simulink model "RR_Target_sim"  (R2023b)
settings: Solver=VariableStepAuto  StartTime=0.0  StopTime=100  RelTol=1e-3
values from neighbouring files (symbols this model uses):
  RR_Aero_Aoa = [-40 -20 -10 -5 0 5 10 20 40]    [RR.mat]    (also in aero.m = [-40.0, -20.0, -10.0, -5.0, 0.0, 5.0, 10.0, 20.0, 40.0])
  RR_Aero_CD = [0.682566420597 0.618503123563 0.559439658146 0.524132967178 0.485737326161 0.447874599784 0.410140259349 0.344355457301 0.271986762452 0.285740001736 0.220860646778 0.173194791928 ... (405 elements, 9x9x5)]    [RR.mat]    (also in aero.m = flip([0.271986762452 0.048967807354 0.024623797928 0.0311930)
  RR_Aero_CL = [-1.32787481318 -1.28000797148 -1.22978921447 -1.19580936529 -1.15925228344 -1.11732991534 -1.07321949156 -0.982213833372 -0.840672452343 -1.01110225062 -0.901800471345 -0.804191382013 ... (405 elements, 9x9x5)]    [RR.mat]    (also in aero.m = flip([-0.840672452343 -0.271053660865 0.064194032020 0.23384)
  RR_Aero_CMy = [0.261776710059 0.227892723507 0.194122810948 0.17203964717 0.149197278338 0.123782621534 0.09809104025 0.048156954183 -0.022673613914 0.230490752369 0.172298182326 0.122095577928 ... (405 elements, 9x9x5)]    [RR.mat]    (also in aero.m = flip([-0.022673613914 -0.123256713392 -0.153636001960 -0.164)
  RR_Aero_Elevons = [-40 -20 -10 -5 0 5 10 20 40]    [RR.mat]    (also in aero.m = [-40.0, -20.0, -10.0, -5.0, 0.0, 5.0, 10.0, 20.0, 40.0])
  RR_Aero_Mach = [0.01 0.1 0.2 0.5 0.9]    [RR.mat]    (also in aero.m = [0.01, 0.1, 0.2, 0.5, 0.9])
  RR_Iyy = 4.432    [RR.mat]
  RR_Motors_Thrust = [4.04656097579 98.9159349639]    [RR.mat]
  RR_Motors_Thrust_Alt_Lut = [0 10000 20000 30000]    [RR.mat]
  RR_Motors_Thrust_Pct_Lut = [1 0.705882352941 0.470588235294 0.352941176471]    [RR.mat]
  RR_Span = 3.6    [RR.mat]
  RR_X_CG = 0.732425    [RR.mat]
  RR_X_NP = 0.9170209    [RR.mat]
  SIM_G = 32.174    [RR.mat]    (also in RR_Forces_ws.m = G; RR_Pitch_ws.m = G; RR_Target_sim_ws.m = G; RR_Target_ws.m = G)
  SIM_INITAL_ALT = -1000    [RR.mat]    (also in RR_Forces_ws.m; RR_Pitch_ws.m = 0; RR_Target_sim_ws.m = 0; RR_Target_ws.m = 0)
  SIM_INITAL_PITCH = 90    [RR_Target_sim_ws.m]    (also in RR_Target_ws.m)
  SIM_INITAL_VEL = 750    [RR.mat]    (also in RR_Forces_ws.m; RR_Pitch_ws.m = 11; RR_Target_sim_ws.m = 15; RR_Target_ws.m = 15)
  SIM_TARGET_ALT = -20000    [RR_Target_sim_ws.m]    (also in RR_Target_ws.m)
  SIM_TARGET_VEL = convvel(290,'kts','ft/s')    [RR_Target_sim_ws.m]    (also in RR_Target_ws.m)
  SIM_TARGET_X = 10    [RR_Target_sim_ws.m]    (also in RR_Target_ws.m = 5000)
undefined symbols (not defined in the file or in its folder): deg, rad, s
libraries: simulink_extras x4, aerolibasang x2, simulink x1, slpidlib x1, aerolib6dof2 x1, aerolibconvert2 x1, aerolibadyn x1, aerolibatmos2 x1, aerolibguid x1, vrlib x1
settings Model: Creator=jrighetti  LastModifiedBy=jrighetti

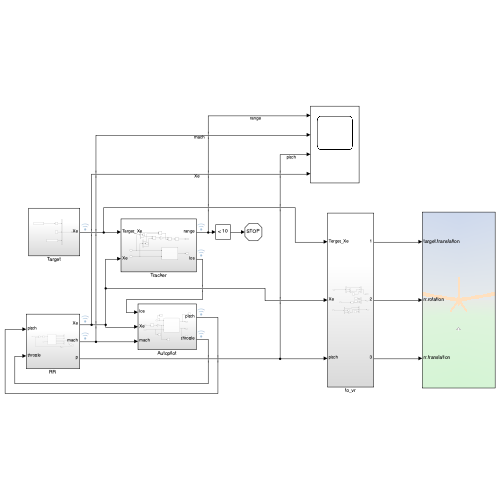
[thumbnail: Simulink's stored preview of the top-level diagram]
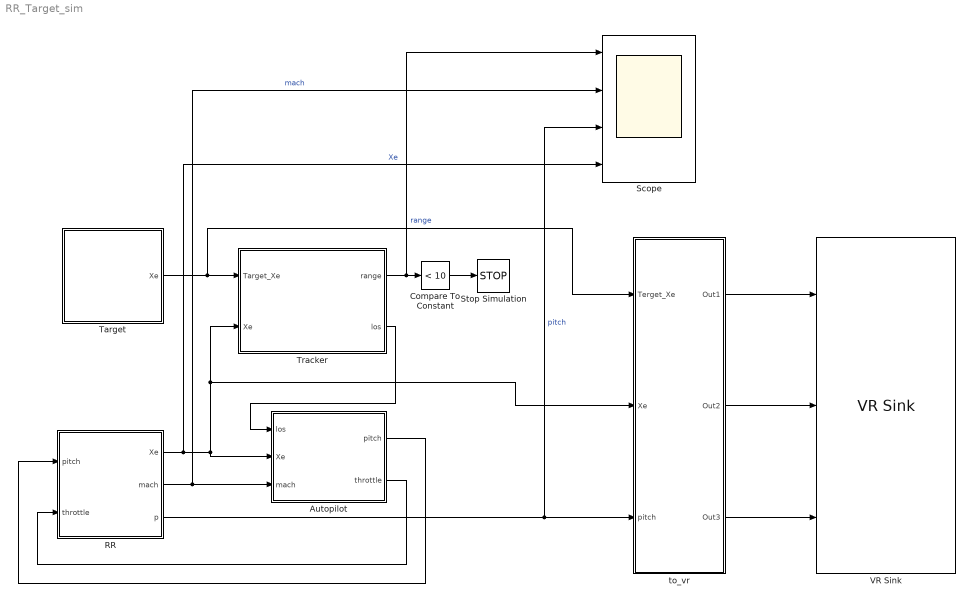
== system RR_Target_sim ==
  Autopilot : Subsystem
  Compare To Constant : simulink/Logic and Bit Operations/Compare To Constant  relop=<  const=10  OutDataTypeStr=boolean
  RR : Subsystem
  Scope : Scope  NumInputPorts=4
  Stop Simulation : Stop
  Target : Subsystem
  Tracker : Subsystem
  VR Sink : vrlib/VR Sink  InstantiateOnLoad=on  SampleTime=-1  ViewEnable=on  RemoteChange=off  RemoteView=off  FieldsWritten=target.translation.3.1.1.double#rr.rotation.4.1.1.double#rr.translation.3.1.1.double  WorldFileName=RR_Target_sim.x3d  AutoView=on  VideoDimensions=[]  AllowVariableSize=off
  to_vr : Subsystem
  wires:
  Target/1(Xe) -> to_vr/1(Terget_Xe), Tracker/1(Target_Xe)
  Compare To Constant/1 -> Stop Simulation/1
  Tracker/1(range) -> Scope/1, Compare To Constant/1  "range"
  RR/1(Xe) -> Scope/4, to_vr/2(Xe), Tracker/2(Xe), Autopilot/2(Xe)  "Xe"
  Tracker/2(los) -> Autopilot/1(los)
  RR/2(mach) -> Scope/2, Autopilot/3(mach)  "mach"
  Autopilot/1(pitch) -> RR/1(pitch)
  Autopilot/2(throttle) -> RR/2(throttle)
  RR/3(p) -> Scope/3, to_vr/3(pitch)  "pitch"
  to_vr/1(Out1) -> VR Sink/1
  to_vr/2(Out2) -> VR Sink/2
  to_vr/3(Out3) -> VR Sink/3

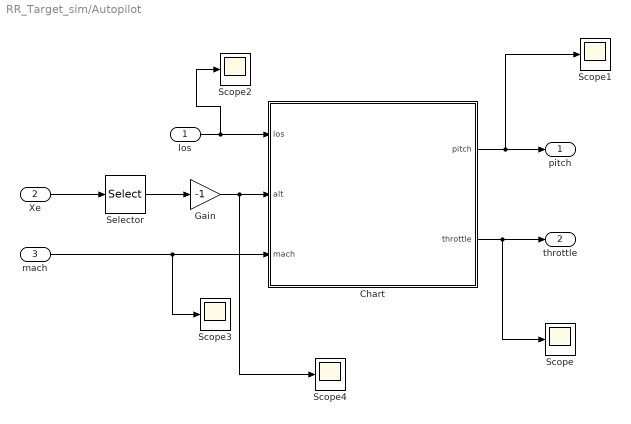
== system RR_Target_sim/Autopilot ==
  los : Inport
  Xe : Inport  Port=2
  mach : Inport  Port=3
  Chart : Stateflow chart  TreatAsAtomicUnit=on
  Gain : Gain  Gain=-1
  Scope{,1..4} (5 alike) : Scope
  Selector : Selector  InputPortWidth=3  IndexOptions=Index vector (dialog)  Indices=3  OutputSizes=1
  pitch : Outport
  throttle : Outport  Port=2
  wires:
  los/1 -> Scope2/1, Chart/1(los)
  Xe/1 -> Selector/1
  mach/1 -> Scope3/1, Chart/3(mach)
  Chart/2(throttle) -> Scope/1, throttle/1
  Selector/1 -> Gain/1
  Gain/1 -> Scope4/1, Chart/2(alt)
  Chart/1(pitch) -> Scope1/1, pitch/1

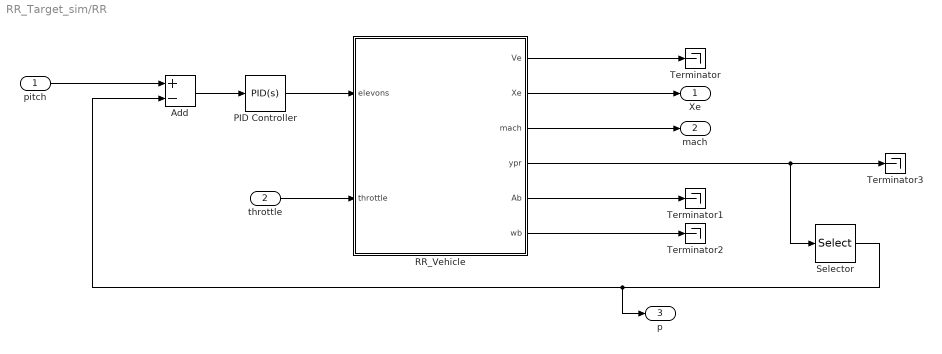
== system RR_Target_sim/RR ==
  pitch : Inport
  throttle : Inport  Port=2
  Add : Sum  Inputs=+-
  PID Controller : slpidlib/PID Controller  Controller=PID  Form=Parallel  TimeDomain=Continuous-time  UseExternalTs=off  SampleTime=-1  IntegratorMethod=Forward Euler  FilterMethod=Forward Euler  ControllerParametersSource=internal  P=0.454470686879052  I=0.32028398620468  UseKiTs=off  D=0.0230057100877012  N=14.587296267084  UseFilter=on  TunerSelectOption=Transfer Function Based (PID Tuner App)  InitialConditionSource=internal  InitialConditionForIntegrator=0  InitialConditionForFilter=0  DifferentiatorICPrevScaledInput=0  ExternalReset=none  TrackingMode=off  Kt=1  LimitOutput=off  SatLimitsSource=internal  UpperSaturationLimit=inf  LowerSaturationLimit=-inf  LinearizeAsGain=on  AntiWindupMode=none  Kb=1  LimitIntegrator=off  UpperIntegratorSaturationLimit=inf  LowerIntegratorSaturationLimit=-inf  POutMin=[]  POutMax=[]  IOutMin=[]  IOutMax=[]  DOutMin=[]  DOutMax=[]  NOutMin=[]  NOutMax=[]  SumOutMin=[]  SumOutMax=[]  SaturationOutMin=[]  SaturationOutMax=[]  PParamMin=[]  PParamMax=[]  IParamMin=[]  IParamMax=[]  DParamMin=[]  DParamMax=[]  NParamMin=[]  NParamMax=[]  KbParamMin=[]  KbParamMax=[]  KtParamMin=[]  KtParamMax=[]  KbOutMin=[]  KbOutMax=[]  KtOutMin=[]  KtOutMax=[]  IntegratorOutMin=[]  IntegratorOutMax=[]  FilterOutMin=[]  FilterOutMax=[]  SumI1OutMin=[]  SumI1OutMax=[]  SumI2OutMin=[]  SumI2OutMax=[]  SumI3OutMin=[]  SumI3OutMax=[]  SumI4OutMin=[]  SumI4OutMax=[]  SumDOutMin=[]  SumDOutMax=[]  DifferentiatorOutMin=[]  DifferentiatorOutMax=[]  FilterDiffOutCoefMin=[]  FilterDiffOutCoefMax=[]  ReciprocalOutMin=[]  ReciprocalOutMax=[]  SumDenOutMin=[]  SumDenOutMax=[]  SumNumOutMin=[]  SumNumOutMax=[]  DivideOutMin=[]  DivideOutMax=[]  UdiffTsProdOutMin=[]  UdiffTsProdOutMax=[]  NTsProdOutMin=[]  NTsProdOutMax=[]  UintegralTsProdOutMin=[]  UintegralTsProdOutMax=[]  UngainTsProdOutMin=[]  UngainTsProdOutMax=[]  ClampingZeroOutDataTypeStr=Inherit: Inherit via back propagation  ClampingZeroOutMin=[]  ClampingZeroOutMax=[]  FilterDenConstantOutDataTypeStr=Inherit: Inherit via back propagation  FilterDenConstantOutMin=[]  FilterDenConstantOutMax=[]  PCopyOutDataTypeStr=Inherit: Inherit via back propagation  PCopyOutMin=[]  PCopyOutMax=[]  NCopyOutDataTypeStr=Inherit: Inherit via back propagation  NCopyOutMin=[]  NCopyOutMax=[]  IntegratorContinuousStateAttributes=''  IntegratorStateMustResolveToSignalObject=off  IntegratorRTWStateStorageClass=Auto  FilterContinuousStateAttributes=''  FilterStateMustResolveToSignalObject=off  FilterRTWStateStorageClass=Auto  ParallelPVariant=InternalParameters  IdealPVariant=Disabled  IVariant=InternalParameters  DVariant=InternalParameters  IntegratorVariant=Continuous  SatVariant=Disabled  AWVariant=Passthrough  PCopyVariant=Disabled  TRVariant=Disabled  FdbkBlocksVariant=Forward  IdealPFdbkVariant=Disabled  SatFdbkVariant=Disabled  DerivativeFilterVariant=ContFilter  NVariant=InternalParameters  NCopyVariant=Disabled  FilterICVariant=InternalICsFilter  IntegratorICVariant=InternalICs  ExternalResetVariant=Disabled  TRSumVariant=Passthrough  SumFdbkVariant=Disabled  SumVariant=Sum_PID  TsampFilterVariant=InternalTs  TsampNgainVariant=Passthrough  TsampIntegralVariant=Disabled_SignalSpec  ExternalSaturationOutDataTypeStr=Inherit: Same as second input
  RR_Vehicle : Subsystem
  Selector : Selector  InputPortWidth=3  IndexOptions=Index vector (dialog)  Indices=2  OutputSizes=1
  Terminator{,1..3} (4 alike) : Terminator
  Xe : Outport
  mach : Outport  Port=2
  p : Outport  Port=3
  wires:
  RR_Vehicle/2(Xe) -> Xe/1
  pitch/1 -> Add/1
  PID Controller/1 -> RR_Vehicle/1(elevons)
  Selector/1 -> p/1, Add/2
  RR_Vehicle/4(ypr) -> Terminator3/1, Selector/1
  RR_Vehicle/6(wb) -> Terminator2/1
  RR_Vehicle/5(Ab) -> Terminator1/1
  Add/1 -> PID Controller/1
  throttle/1 -> RR_Vehicle/2(throttle)
  RR_Vehicle/3(mach) -> mach/1
  RR_Vehicle/1(Ve) -> Terminator/1

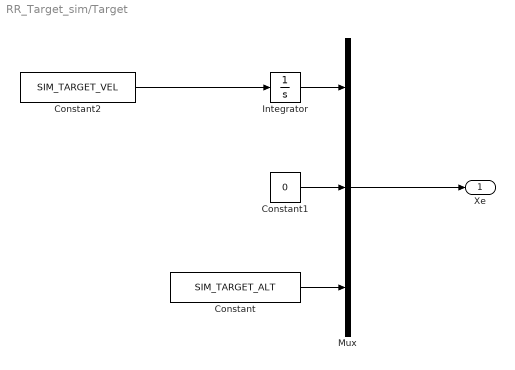
== system RR_Target_sim/Target ==
  Constant : Constant  Value=SIM_TARGET_ALT
  Constant1 : Constant  Value=0
  Constant2 : Constant  Value=SIM_TARGET_VEL
  Integrator : Integrator  InitialCondition=SIM_TARGET_X
  Mux : Mux  Inputs=3
  Xe : Outport
  wires:
  Integrator/1 -> Mux/1
  Mux/1 -> Xe/1
  Constant/1 -> Mux/3
  Constant1/1 -> Mux/2
  Constant2/1 -> Integrator/1

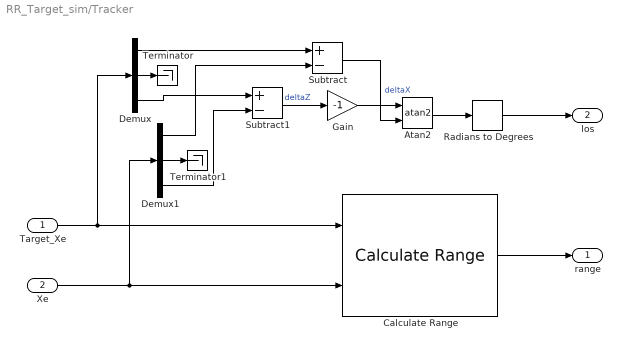
== system RR_Target_sim/Tracker ==
  Target_Xe : Inport
  Xe : Inport  Port=2
  Atan2 : Trigonometry  Operator=atan2
  Calculate Range : aerolibguid/Calculate Range
  Demux : Demux  Outputs=3
  Demux1 : Demux  Outputs=3
  Gain : Gain  Gain=-1
  Radians to Degrees : simulink_extras/Transformations/Radians to Degrees
  Subtract : Sum  Inputs=+-
  Subtract1 : Sum  Inputs=+-
  Terminator : Terminator
  Terminator1 : Terminator
  range : Outport
  los : Outport  Port=2
  wires:
  Subtract/1 -> Atan2/2  "deltaX"
  Subtract1/1 -> Gain/1  "deltaZ"
  Calculate Range/1 -> range/1
  Radians to Degrees/1 -> los/1
  Atan2/1 -> Radians to Degrees/1
  Xe/1 -> Calculate Range/2, Demux1/1
  Target_Xe/1 -> Demux/1, Calculate Range/1
  Demux/1 -> Subtract/1
  Demux1/1 -> Subtract/2
  Demux/3 -> Subtract1/1
  Demux1/3 -> Subtract1/2
  Demux/2 -> Terminator/1
  Demux1/2 -> Terminator1/1
  Gain/1 -> Atan2/1

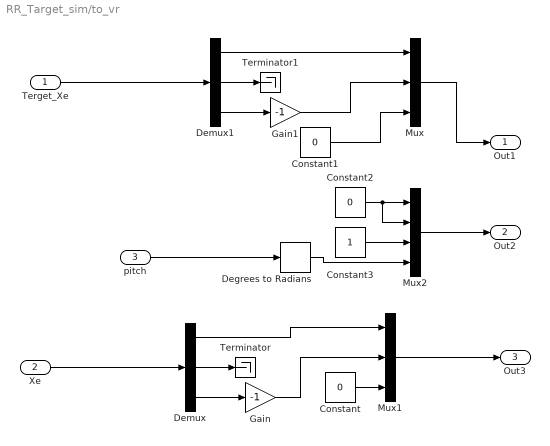
== system RR_Target_sim/to_vr ==
  Terget_Xe : Inport
  Xe : Inport  Port=2
  pitch : Inport  Port=3
  Constant : Constant  Value=0
  Constant1 : Constant  Value=0
  Constant2 : Constant  Value=0
  Constant3 : Constant
  Degrees to Radians : simulink_extras/Transformations/Degrees to Radians
  Demux : Demux  Outputs=3
  Demux1 : Demux  Outputs=3
  Gain : Gain  Gain=-1
  Gain1 : Gain  Gain=-1
  Mux : Mux  Inputs=3
  Mux1 : Mux  Inputs=3
  Mux2 : Mux
  Terminator : Terminator
  Terminator1 : Terminator
  Out1 : Outport
  Out2 : Outport  Port=2
  Out3 : Outport  Port=3
  wires:
  Mux1/1 -> Out3/1
  Degrees to Radians/1 -> Mux2/4
  Demux1/2 -> Terminator1/1
  Demux1/1 -> Mux/1
  Demux/2 -> Terminator/1
  Constant3/1 -> Mux2/3
  Constant1/1 -> Mux/3
  Demux/3 -> Gain/1
  Demux/1 -> Mux1/1
  Mux2/1 -> Out2/1
  Gain1/1 -> Mux/2
  Constant/1 -> Mux1/3
  Terget_Xe/1 -> Demux1/1
  Xe/1 -> Demux/1
  Gain/1 -> Mux1/2
  Mux/1 -> Out1/1
  Demux1/3 -> Gain1/1
  pitch/1 -> Degrees to Radians/1
  Constant2/1 -> Mux2/2, Mux2/1

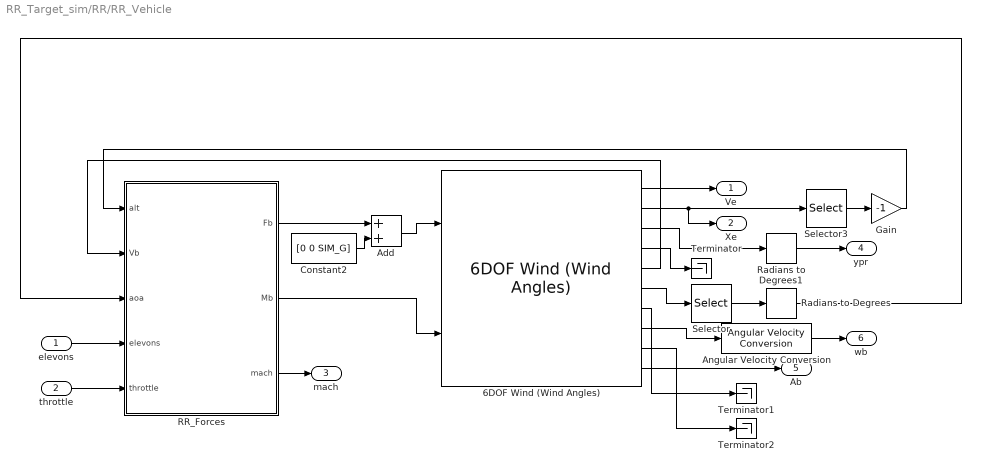
== system RR_Target_sim/RR/RR_Vehicle ==
  elevons : Inport
  throttle : Inport  Port=2
  6DOF Wind (Wind Angles) : aerolib6dof2/6DOF Wind (Wind Angles)  units=English (Velocity in ft/s)  mtype=Fixed  rep=Wind Angles  xme_0=[0 0 SIM_INITAL_ALT]  Vm_0=[SIM_INITAL_VEL 0 0]  wind_0=[0 deg2rad(SIM_INITAL_PITCH) 0]  pm_0=[0 0 0]  mass_0=RR_Total_Mass  mass_e=RR_Total_Mass  mass_f=RR_Total_Dry_Mass  inertia=diag([1 RR_Iyy 1])  inertia_e=diag([1 RR_Iyy 1])  inertia_f=diag([1 RR_Iyy 1])*0.75  vre_flag=on  abi_flag=off  xme_statename=''  Vm_statename=''  alpha_statename=''  beta_statename=''  wind_statename=''  quat_statename=''  pm_statename=''  mass_statename=''
  Add : Sum
  Angular Velocity Conversion : aerolibconvert2/Angular Velocity Conversion  IU=rad/s  OU=deg/s
  Constant2 : Constant  Value=[0 0 SIM_G]
  Gain : Gain  Gain=-1
  RR_Forces : Subsystem
  Radians to Degrees : simulink_extras/Transformations/Radians to Degrees
  Radians to Degrees1 : simulink_extras/Transformations/Radians to Degrees
  Selector : Selector  InputPortWidth=2  IndexOptions=Index vector (dialog)  Indices=1  OutputSizes=1
  Selector3 : Selector  InputPortWidth=3  IndexOptions=Index vector (dialog)  Indices=3  OutputSizes=1
  Terminator : Terminator
  Terminator1 : Terminator
  Terminator2 : Terminator
  Ve : Outport
  Xe : Outport  Port=2
  mach : Outport  Port=3
  ypr : Outport  Port=4
  Ab : Outport  Port=5
  wb : Outport  Port=6
  wires:
  throttle/1 -> RR_Forces/5(throttle)
  Selector3/1 -> Gain/1
  Radians to Degrees/1 -> RR_Forces/3(aoa)
  6DOF Wind (Wind Angles)/3 -> Radians to Degrees1/1
  6DOF Wind (Wind Angles)/2 -> Xe/1, Selector3/1
  Gain/1 -> RR_Forces/1(alt)
  6DOF Wind (Wind Angles)/6 -> Selector/1
  Selector/1 -> Radians to Degrees/1
  6DOF Wind (Wind Angles)/5 -> RR_Forces/2(Vb)
  RR_Forces/1(Fb) -> Add/1
  RR_Forces/2(Mb) -> 6DOF Wind (Wind Angles)/2
  RR_Forces/3(mach) -> mach/1
  Radians to Degrees1/1 -> ypr/1
  Add/1 -> 6DOF Wind (Wind Angles)/1
  6DOF Wind (Wind Angles)/1 -> Ve/1
  Constant2/1 -> Add/2
  6DOF Wind (Wind Angles)/4 -> Terminator/1
  6DOF Wind (Wind Angles)/10 -> Ab/1
  elevons/1 -> RR_Forces/4(elevons)
  6DOF Wind (Wind Angles)/8 -> Angular Velocity Conversion/1
  6DOF Wind (Wind Angles)/7 -> Terminator1/1
  6DOF Wind (Wind Angles)/9 -> Terminator2/1
  Angular Velocity Conversion/1 -> wb/1

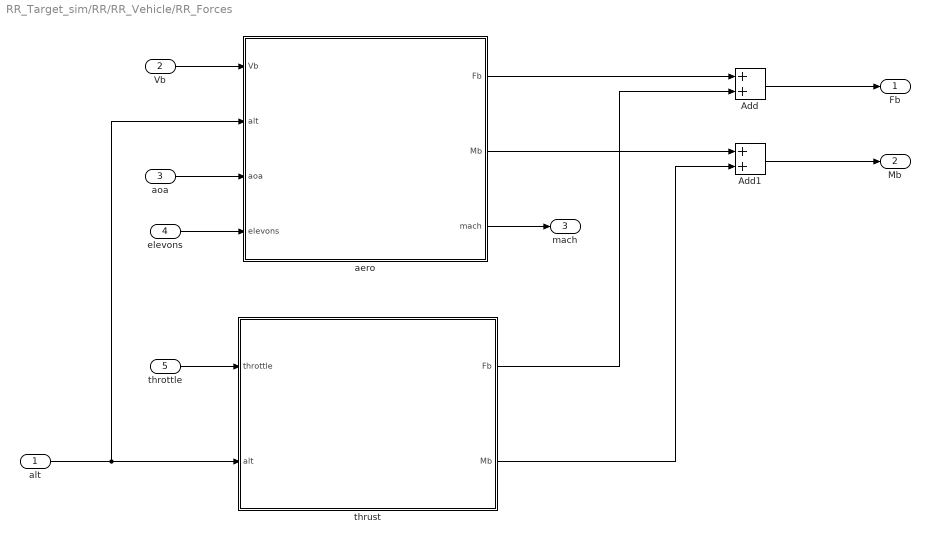
== system RR_Target_sim/RR/RR_Vehicle/RR_Forces ==
  alt : Inport
  Vb : Inport  Port=2
  aoa : Inport  Port=3
  elevons : Inport  Port=4
  throttle : Inport  Port=5
  Add : Sum
  Add1 : Sum
  aero : Subsystem
  thrust : Subsystem
  Fb : Outport
  Mb : Outport  Port=2
  mach : Outport  Port=3
  wires:
  alt/1 -> aero/2(alt), thrust/2(alt)
  Vb/1 -> aero/1(Vb)
  aoa/1 -> aero/3(aoa)
  elevons/1 -> aero/4(elevons)
  throttle/1 -> thrust/1(throttle)
  aero/1(Fb) -> Add/1
  thrust/1(Fb) -> Add/2
  Add/1 -> Fb/1
  aero/2(Mb) -> Add1/1
  thrust/2(Mb) -> Add1/2
  Add1/1 -> Mb/1
  aero/3(mach) -> mach/1

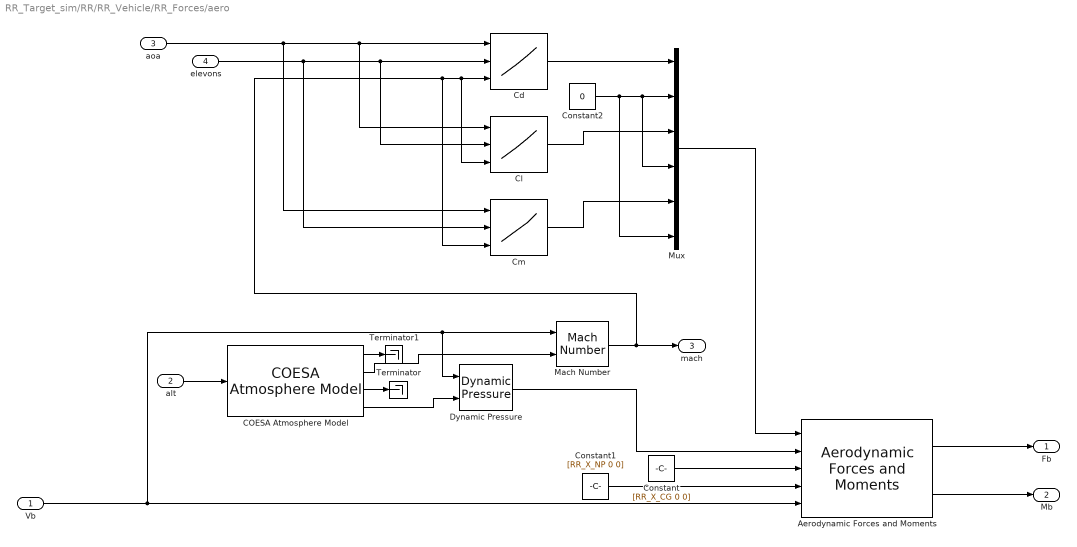
== system RR_Target_sim/RR/RR_Vehicle/RR_Forces/aero ==
  Vb : Inport
  alt : Inport  Port=2
  aoa : Inport  Port=3
  elevons : Inport  Port=4
  "Aerodynamic Forces and Moments " : aerolibadyn/Aerodynamic Forces and Moments   inputAxes=Wind  outputForceAxes=Body  outputMomentAxes=Body  S=RR_AERO_S  b=RR_Span  cbar=RR_AERO_CORD
  COESA Atmosphere Model : aerolibatmos2/COESA Atmosphere Model  units=English (Velocity in ft/s)  spec=1976 COESA-extended U.S. Standard Atmosphere  model=Profile  profile_var=High temperature  profile_percent=1%  profile_alt=5 km (16404 ft)  envelope_var=High temperature  envelope_percent=1%  action=Warning
  Cd : Lookup_n-D  NumberOfTableDimensions=3  BreakpointsForDimension1=RR_Aero_Aoa  BreakpointsForDimension2=RR_Aero_Elevons  BreakpointsForDimension3=RR_Aero_Mach  BreakpointsForDimension1DataTypeStr=Inherit: Inherit from 'Breakpoint data'  Table=RR_Aero_CD  TableDataTypeStr=Inherit: Inherit from 'Table data'  InternalRulePriority=Speed  RndMeth=Simplest
      settings: InputPortMap=u0,u1,u2
  Cl : Lookup_n-D  NumberOfTableDimensions=3  BreakpointsForDimension1=RR_Aero_Aoa  BreakpointsForDimension2=RR_Aero_Elevons  BreakpointsForDimension3=RR_Aero_Mach  Table=RR_Aero_CL  DiagnosticForOutOfRangeInput=Warning  InternalRulePriority=Speed  RndMeth=Simplest
      settings: InputPortMap=u0,u1,u2
  Cm : Lookup_n-D  NumberOfTableDimensions=3  BreakpointsForDimension1=RR_Aero_Aoa  BreakpointsForDimension2=RR_Aero_Elevons  BreakpointsForDimension3=RR_Aero_Mach  Table=RR_Aero_CMy  DiagnosticForOutOfRangeInput=Warning  InternalRulePriority=Speed  RndMeth=Simplest
      settings: InputPortMap=u0,u1,u2
  Constant : Constant  Value=[RR_X_CG 0 0]
  Constant1 : Constant  Value=[RR_X_NP 0 0]
  Constant2 : Constant  Value=0
  Dynamic Pressure : aerolibasang/Dynamic Pressure
  Mach Number : aerolibasang/Mach Number
  Mux : Mux  Inputs=6
  Terminator : Terminator
  Terminator1 : Terminator
  Fb : Outport
  Mb : Outport  Port=2
  mach : Outport  Port=3
  wires:
  Dynamic Pressure/1 -> "Aerodynamic Forces and Moments "/2
  Constant2/1 -> Mux/6, Mux/4, Mux/2
  alt/1 -> COESA Atmosphere Model/1
  "Aerodynamic Forces and Moments "/1 -> Fb/1
  COESA Atmosphere Model/2 -> Mach Number/2
  COESA Atmosphere Model/3 -> Terminator/1
  Constant/1 -> "Aerodynamic Forces and Moments "/3
  COESA Atmosphere Model/4 -> Dynamic Pressure/2
  "Aerodynamic Forces and Moments "/2 -> Mb/1
  elevons/1 -> Cm/2, Cl/2, Cd/2
  Mach Number/1 -> mach/1, Cm/3, Cl/3, Cd/3
  Mux/1 -> "Aerodynamic Forces and Moments "/1
  Cl/1 -> Mux/3
  Constant1/1 -> "Aerodynamic Forces and Moments "/4
  aoa/1 -> Cm/1, Cl/1, Cd/1
  Cd/1 -> Mux/1
  COESA Atmosphere Model/1 -> Terminator1/1
  Cm/1 -> Mux/5
  Vb/1 -> "Aerodynamic Forces and Moments "/5, Dynamic Pressure/1, Mach Number/1

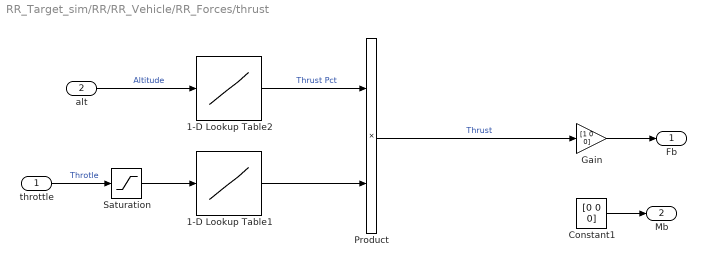
== system RR_Target_sim/RR/RR_Vehicle/RR_Forces/thrust ==
  throttle : Inport
  alt : Inport  Port=2
  1-D Lookup Table1 : Lookup_n-D  NumberOfTableDimensions=1  BreakpointsForDimension1=[0,1]  Table=RR_Motors_Thrust  InternalRulePriority=Speed  RndMeth=Simplest
  1-D Lookup Table2 : Lookup_n-D  NumberOfTableDimensions=1  BreakpointsForDimension1=RR_Motors_Thrust_Alt_Lut  Table=RR_Motors_Thrust_Pct_Lut  InternalRulePriority=Speed  RndMeth=Simplest
  Constant1 : Constant  Value=[0 0 0]
  Gain : Gain  Gain=[1 0 0]
  Product : Product
  Saturation : Saturate  UpperLimit=1.0  LowerLimit=0.0
  Fb : Outport
  Mb : Outport  Port=2
  wires:
  throttle/1 -> Saturation/1  "Throtle"
  alt/1 -> 1-D Lookup Table2/1  "Altitude"
  1-D Lookup Table2/1 -> Product/1  "Thrust Pct"
  1-D Lookup Table1/1 -> Product/2
  Saturation/1 -> 1-D Lookup Table1/1
  Product/1 -> Gain/1  "Thrust"
  Gain/1 -> Fb/1
  Constant1/1 -> Mb/1

== stateflow chart RR_Target_sim/Autopilot/Chart ==
  state launch
    throttle=1.0;
    pitch=90.0;
  state cruise
    throttle=0.75;
    pitch=45.0;
  state target
    throttle=1.0;
    pitch=los;
  (default) -> launch
  cruise -> target : [mach>0.5]
  launch -> cruise : [alt>2000]
  data: los input; alt input; mach input; pitch output; throttle output
